simulink model "GalacticSoupComplianceGate"  (R2026a)
settings: Solver=VariableStepAuto  StopTime=1
model workspace (MAT data in the model file):
  AUTO_FLOOR = 0.8
  COST_CAP = 2000
  GRAV_FLOOR = 12
  MASS_CAP = 15000
  OPS_CAP = 5
  POWER_CAP = 500
  THR_FLOOR = 200
  VOL_CAP = 400
settings Model: Creator=sarah  LastModifiedBy=sarah

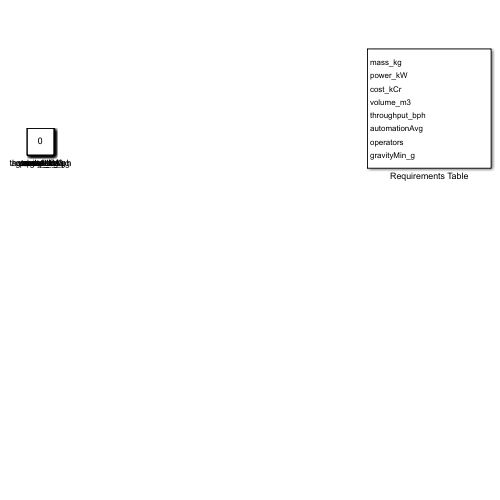
[thumbnail: Simulink's stored preview of the top-level diagram]
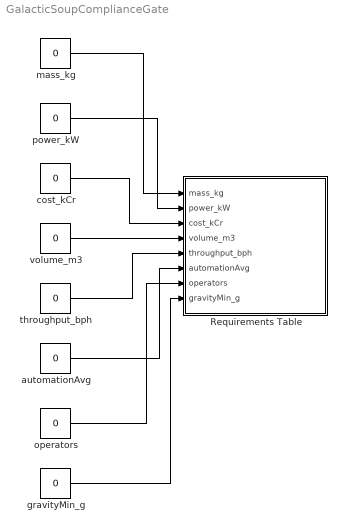
== system GalacticSoupComplianceGate ==
  Requirements Table : Requirements Table  TreatAsAtomicUnit=on
  automationAvg : Constant  Value=0
  cost_kCr : Constant  Value=0
  gravityMin_g : Constant  Value=0
  mass_kg : Constant  Value=0
  operators : Constant  Value=0
  power_kW : Constant  Value=0
  throughput_bph : Constant  Value=0
  volume_m3 : Constant  Value=0
  wires:
  mass_kg/1 -> Requirements Table/1(mass_kg)
  power_kW/1 -> Requirements Table/2(power_kW)
  cost_kCr/1 -> Requirements Table/3(cost_kCr)
  volume_m3/1 -> Requirements Table/4(volume_m3)
  throughput_bph/1 -> Requirements Table/5(throughput_bph)
  automationAvg/1 -> Requirements Table/6(automationAvg)
  operators/1 -> Requirements Table/7(operators)
  gravityMin_g/1 -> Requirements Table/8(gravityMin_g)

== stateflow chart GalacticSoupComplianceGate/Requirements Table ==
  settings: updateMethod=DISCRETE  sampleTime=1
  (default) -> (junction 1073741909)
  (junction 1073741909) -> (junction 1073741910) : {
      | % SF_REQ_REV_09
      | }
  (junction 1073741910) -> (junction 1073741912) : {
      | % ExcEvals:
      | % PriEvals:
      | }
  (junction 1073741912) -> (junction 1073741914) : {
      | % HEADER_ASSIGNMENTS
      |
      | }
  (junction 1073741914) -> (junction 1073741916) : {
      | % START_A_4
      | }
  (junction 1073741916) -> (junction 1073741918) : {
      | }
  (junction 1073741918) -> (junction 1073741920)
  (junction 1073741920) -> (junction 1073741922) : {
      | }
  (junction 1073741922) -> (junction 1073741924) : {
      | % END_A_4
      | }
  (junction 1073741924) -> (junction 1073741926) : {
      | % START_R_1
      | }
  (junction 1073741926) -> (junction 1073741928) : {
      | }
  (junction 1073741928) -> (junction 1073741930) : {
      |
      |
      | }
  (junction 1073741930) -> (junction 1073741932) : {
      | }
  (junction 1073741932) -> (junction 1073741934) : {
      | % END_R_1
      | }
  (junction 1073741934) -> (junction 1073741954) : {
      | % START_R_7
      | }
  (junction 1073741954) -> (junction 1073741956) : {
      | }
  (junction 1073741956) -> (junction 1073741958) : {
      | reqtable_postcondition((mass_kg <= MASS_CAP), 'R:2');
      |
      |
      | }
  (junction 1073741958) -> (junction 1073741960) : {
      | }
  (junction 1073741960) -> (junction 1073741962) : {
      | % END_R_7
      | }
  (junction 1073741962) -> (junction 1073741966) : {
      | % START_R_10
      | }
  (junction 1073741966) -> (junction 1073741968) : {
      | }
  (junction 1073741968) -> (junction 1073741970) : {
      | reqtable_postcondition((power_kW <= POWER_CAP), 'R:3');
      |
      |
      | }
  (junction 1073741970) -> (junction 1073741972) : {
      | }
  (junction 1073741972) -> (junction 1073741974) : {
      | % END_R_10
      | }
  (junction 1073741974) -> (junction 1073741978) : {
      | % START_R_13
      | }
  (junction 1073741978) -> (junction 1073741980) : {
      | }
  (junction 1073741980) -> (junction 1073741982) : {
      | reqtable_postcondition((cost_kCr <= COST_CAP), 'R:4');
      |
      |
      | }
  (junction 1073741982) -> (junction 1073741984) : {
      | }
  (junction 1073741984) -> (junction 1073741986) : {
      | % END_R_13
      | }
  (junction 1073741986) -> (junction 1073741990) : {
      | % START_R_16
      | }
  (junction 1073741990) -> (junction 1073741992) : {
      | }
  (junction 1073741992) -> (junction 1073741994) : {
      | reqtable_postcondition((volume_m3 <= VOL_CAP), 'R:5');
      |
      |
      | }
  (junction 1073741994) -> (junction 1073741996) : {
      | }
  (junction 1073741996) -> (junction 1073741998) : {
      | % END_R_16
      | }
  (junction 1073741998) -> (junction 1073742002) : {
      | % START_R_19
      | }
  (junction 1073742002) -> (junction 1073742004) : {
      | }
  (junction 1073742004) -> (junction 1073742006) : {
      | reqtable_postcondition((throughput_bph >= THR_FLOOR), 'R:6');
      |
      |
      | }
  (junction 1073742006) -> (junction 1073742008) : {
      | }
  (junction 1073742008) -> (junction 1073742010) : {
      | % END_R_19
      | }
  (junction 1073742010) -> (junction 1073742014) : {
      | % START_R_22
      | }
  (junction 1073742014) -> (junction 1073742016) : {
      | }
  (junction 1073742016) -> (junction 1073742018) : {
      | reqtable_postcondition((automationAvg >= AUTO_FLOOR), 'R:7');
      |
      |
      | }
  (junction 1073742018) -> (junction 1073742020) : {
      | }
  (junction 1073742020) -> (junction 1073742022) : {
      | % END_R_22
      | }
  (junction 1073742022) -> (junction 1073742026) : {
      | % START_R_25
      | }
  (junction 1073742026) -> (junction 1073742028) : {
      | }
  (junction 1073742028) -> (junction 1073742030) : {
      | reqtable_postcondition((operators <= OPS_CAP), 'R:8');
      |
      |
      | }
  (junction 1073742030) -> (junction 1073742032) : {
      | }
  (junction 1073742032) -> (junction 1073742034) : {
      | % END_R_25
      | }
  (junction 1073742034) -> (junction 1073742038) : {
      | % START_R_28
      | }
  (junction 1073742038) -> (junction 1073742040) : {
      | }
  (junction 1073742040) -> (junction 1073742042) : {
      | reqtable_postcondition((gravityMin_g >= GRAV_FLOOR), 'R:9');
      |
      |
      | }
  (junction 1073742042) -> (junction 1073742044) : {
      | }
  (junction 1073742044) -> (junction 1073742046) : {
      | % END_R_28
      | }
  data: mass_kg input double size=1; power_kW input double size=1; cost_kCr input double size=1; volume_m3 input double size=1; throughput_bph input double size=1; automationAvg input double size=1; operators input double size=1; gravityMin_g input double size=1; MASS_CAP parameter double size=1; POWER_CAP parameter double size=1; COST_CAP parameter double size=1; VOL_CAP parameter double size=1; THR_FLOOR parameter double size=1; AUTO_FLOOR parameter double size=1; OPS_CAP parameter double size=1; GRAV_FLOOR parameter double size=1
